simulink model "unstable_system_Linear_MPC"  (R2024b)
settings: configuration reference "unstable_system_config" (kept outside this file)
undefined symbols (not defined in the file): controller_sw
settings Model: DataDictionary=sim_data_unstable_system.sldd  SILPILSystemUnderTest=refmodels  Creator=tshintai  LastModifiedBy=tshintai
settings ConfigSetRef: SourceName=unstable_system_config

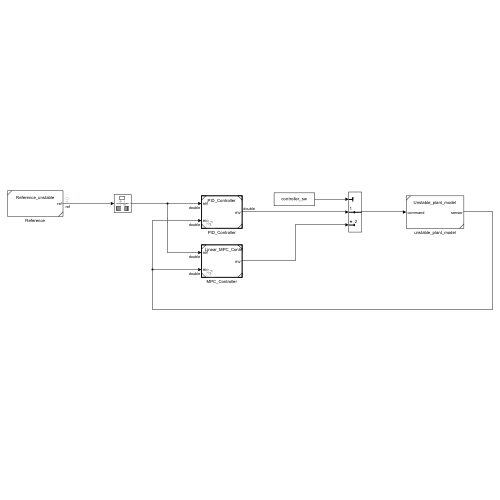
[thumbnail: Simulink's stored preview of the top-level diagram]
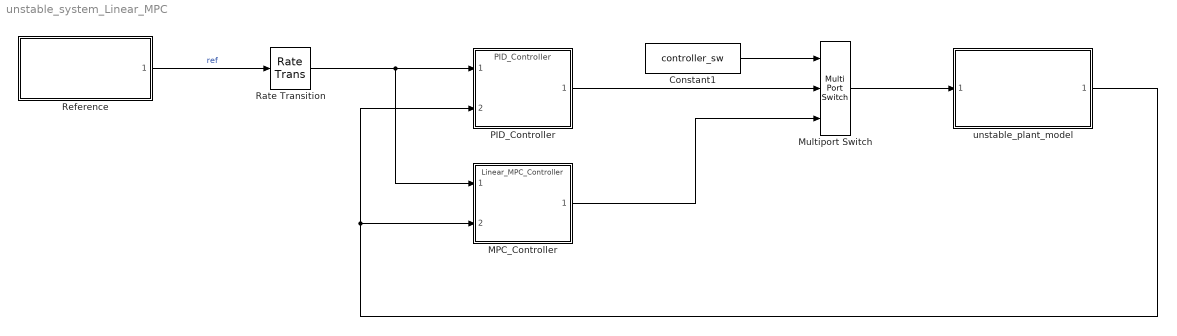
== system unstable_system_Linear_MPC ==
  Constant1 : Constant  Value=controller_sw  OutDataTypeStr=uint32
  MPC_Controller : ModelReference  ModelNameDialog=Linear_MPC_Controller.slx  SimulationMode=Normal  ModelReferenceVersion=8.0
  Multiport Switch : MultiPortSwitch  Inputs=2  DiagnosticForDefault=None  SaturateOnIntegerOverflow=off  InputSameDT=off
  PID_Controller : ModelReference  ModelNameDialog=PID_Controller  SimulationMode=Normal  ModelReferenceVersion=9.0
  Rate Transition : RateTransition  OutPortSampleTime=TimeStep
  Reference : Subsystem  ReferencedSubsystem=Reference_unstable
  unstable_plant_model : Subsystem  ReferencedSubsystem=Unstable_plant_model
  wires:
  PID_Controller/1 -> Multiport Switch/2
  Constant1/1 -> Multiport Switch/1
  Reference/1 -> Rate Transition/1  "ref"
  MPC_Controller/1 -> Multiport Switch/3
  Rate Transition/1 -> MPC_Controller/1, PID_Controller/1
  unstable_plant_model/1 -> PID_Controller/2, MPC_Controller/2
  Multiport Switch/1 -> unstable_plant_model/1
